simulink model "SpeedControlTest_vDemo_TC"  (Simulink 6.6)
settings: Solver=ode4  SolverMode=SingleTasking  StartTime=0.0  StopTime=252  FixedStep=0.01  RelTol=1e-3
InitFcn:
  | tempomat_para
StopFcn:
  | clear;
values from neighbouring files (symbols this model uses):
  A = 1.9    [tempomat_para.m]
  a_Fzg_max = 2    [tempomat_para.m]
  a_Fzg_min = -2    [tempomat_para.m]
  cw = 0.32    [tempomat_para.m]
  gang = [1 2 3 4]    [tempomat_para.m]
  gang_vec = [1 2 3 4]    [tempomat_para.m]
  i_anteil = 5    [tempomat_para.m]
  i_d = 3.42    [tempomat_para.m]
  i_g = [3.91 2.17 1.37 1.00]    [tempomat_para.m]
  lambda_gang = [1.3 1.25  1.17  1.05]    [tempomat_para.m]
  m_Fzg = 1400    [tempomat_para.m]
  M_mot_max = [130 149 163 170 168 166 162 158 150 139 123 80]    [tempomat_para.m]
  M_mot_min = [0 -40]    [tempomat_para.m]
  n_mot0 = 1000    [tempomat_para.m]
  n_mot_max = 1000:500:6500    [tempomat_para.m]
  n_mot_min = [1000 6500]    [tempomat_para.m]
  p_anteil = 100    [tempomat_para.m]
  r_dyn = 0.28    [tempomat_para.m]
  rho = 1.202    [tempomat_para.m]
  t_sch = 0.2    [tempomat_para.m]
  TI = [block '/TI']    [PSTI_callback.m]
  v_Fzg_ms0 = 0    [tempomat_para.m]
undefined symbols (not defined in the file or in its folder): Drossel_mat, getdatatypespecs
libraries: simulink x113, fzgbib x3
(part 3 of 9)

== system SpeedControlTest_vDemo_TC/Validation Functions/R1 Speed Control step response/Maximum overshoot < 5 &  Steady state error < 5/Step response characteristics ==
  Step : Inport
  Step response : Inport  Port=2
  Step response characteristics extraction : Subsystem  mask(Step response feature extraction){gain=1, lowerLim=10, upperLim=90, MOma=0.01*ones(1,100), RelTol=0.0001, MinTime=5, Range=5, sseW=0.01*ones(1,100)}
      mask prompts: gain "System's static gain"; lowerLim "Rise time interval lower limit (in set point %)"; upperLim "Rise time interval upper limit (in set point %)"; MOma "Maximum overshoot moving average weights"; RelTol "Maximum overshoot - Detect constant if no overshoot - Relative Tolerance"; MinTime "Maximum overshoot - Detect constant if no overshoot - Minimum constant time"; Range "Settling time range (in set point %)"; sseW "Steady state error - moving average weights"
      mask help: Extracts four step response feature characteristics. Extraction parameters are shown below.
      mask CallbackString:
      | set_param([gcb '/Static Gain'],'Value',get_param(gcb,'gain'));|set_param([gcb '/Extract rise time/lowerLim'],'Value',get_param(gcb,'lowerLim'));|set_param([gcb '/Extract rise time/upperLim'],'Value',get_param(gcb,'upperLim'));|set_param([gcb '/Extract maximum overshoot/Step response moving average and initial conditions before step/Weighted Moving Average'],'mgainval',get_param(gcb,'MOma'));
      | set_param([gcb '/Extract maximum overshoot/Step response moving average and initial conditions before step/Weighted Moving Average1'],'mgainval',get_param(gcb,'MOma'));|set_param([gcb '/Extract maximum overshoot/Active if signals constant for some specified time/Time since signal constant'],'RT',get_param(gcb,'RelTol'));
      | set_param([gcb '/Extract maximum overshoot/Active if signals constant for some specified time/Time since signal constant1'],'RT',get_param(gcb,'RelTol'));|set_param([gcb '/Extract maximum overshoot/Active if signals constant for some specified time/Min Time'],'Value',get_param(gcb,'MinTime'));|set_param([gcb '/Extract settling time/Set point percent'],'Value',get_param(gcb,'Range'));|set_param([gcb '/Extract steady state error/Weighted Moving Average'],'mgainval',get_param(gcb,'sseW'));
  Step response reset : Subsystem  mask{MT=10, RT=0.0001, MSS=10}
      mask prompts: MT "Minimal time for signals to be constant before a step"; RT "Relative tolerance for constant detection in %"; MSS "Minimal step size for step detection"
      mask CallbackString:
      | if (str2double(get_param(gcb,'MT')) < 0)
      |     error(['Minimal time specified (' get_param(gcb,'MT') ') negative. Please give a non-negative value.']);
      | else
      |     set_param([gcb '/Active if signals constant for some specified time/Min Time'],'Value',get_param(gcb,'MT'));
      | end|if or( (str2double(get_param(gcb,'RT')) < 0), (str2double(get_param(gcb,'RT')) > 100))
      |     error(['Relative tolerance value (' get_param(gcb,'RT') ') out of range. Please give a value between 0 and 100.']);
      | else
      |     set_param([gcb '/Active if signals constant for some specified time/Time since signal constant/Detect constant/Relative tolerance/Relative Tolerance'],'Value',get_param(gcb,'RT'));
      |     set_param([gcb '/Active if signals constant for some specified time/Time since signal constant/Detect constant'],'RT',get_param(gcb,'RT'));
      |     set_param([gcb '/Active if signals constant for some specified time/Time since signal constant'],'RT',get_param(gcb,'RT'));
      |     set_param([gcb '/Active if signals constant for some specified time/Time since signal constant1/Detect constant/Relative tolerance/Relative Tolerance'],'Value',get_param(gcb,'RT'));
      |     set_param([gcb '/Active if signals constant for some specified time/Time since signal constant1/Detect constant'],'RT',get_param(gcb,'RT'));
      |     set_param([gcb '/Active if signals constant for some specified time/Time since signal constant1'],'RT',get_param(gcb,'RT'));
      | end|if (str2double(get_param(gcb,'MSS')) < 0)
      |     error(['Minimal step size specified (' get_param(gcb,'MSS') ') negative. Please give a non-negative value.']);
      | else
      |     set_param([gcb '/Step detection/Min step size'],'Value',get_param(gcb,'MSS'));
      |     set_param([gcb '/Step detection'],'StepSize',get_param(gcb,'MSS'));
      | 
      | end
  Step response trigger : Subsystem  mask(Step response trigger extraction){MinTime=10, RelTol=0.001, MAXsse=5}
      mask prompts: MinTime "Detect constant signals - Minimum constant time"; RelTol "Detect constant signals - Relative Tolerance"; MAXsse "Maximum steady state error for triggering"
      mask help: This block extracts the trigger signals for the four step response characteristics.
      mask CallbackString:
      | set_param([gcb '/Active if signals constant for some specified time/Min Time'],'Value',get_param(gcb,'MinTime'));|set_param([gcb '/Active if signals constant for some specified time/Time since signal constant'],'RT',get_param(gcb,'RelTol'));
      | set_param([gcb '/Active if signals constant for some specified time/Time since signal constant1'],'RT',get_param(gcb,'RelTol'));|set_param([gcb '/Compare To Constant'],'const',get_param(gcb,'MAXsse'));
  R : Outport
  Rise time T : Outport  Port=2  DataType=double
  Overshoot T : Outport  Port=3  DataType=double
  Settling time T : Outport  Port=4  DataType=double
  Steady state error T : Outport  Port=5  DataType=double
  Rise time : Outport  Port=6
  Maximum Overshoot : Outport  Port=7
  Settling time : Outport  Port=8  DataType=double
  Steady state error : Outport  Port=9  DataType=double
  wires:
  Step response reset/1(R) -> R/1, Step response characteristics extraction/1(R)
  Step response characteristics extraction/4(Steady state error) -> Step response trigger/1(Steady state error), Steady state error/1
  Step/1 -> Step response reset/1(Step), Step response characteristics extraction/2(Step)
  Step response/1 -> Step response reset/2(Step response), Step response characteristics extraction/3(Step response), Step response trigger/2(Step response)
  Step response characteristics extraction/1(Rise time) -> Rise time/1
  Step response characteristics extraction/3(Settling time) -> Settling time/1
  Step response characteristics extraction/2(Maximum overshoot) -> Maximum Overshoot/1
  Step response trigger/1(Rise time T) -> Rise time T/1
  Step response trigger/2(Overshoot T) -> Overshoot T/1
  Step response trigger/3(Settling time T) -> Settling time T/1
  Step response trigger/4(Steady state error T) -> Steady state error T/1

== system SpeedControlTest_vDemo_TC/Validation Functions/R2 Speed Control velocity restoration time after simple  acceleration or deceleration/CC active + no target & Speed Control active & step of V_Des = |1|  with time periods >= 7s/CC active & no target ==
  Signal : Inport
  Reference : Inport  Port=2
  Abs : Abs
  Abs1 : Abs
  Absolute Tolerance : Constant  Value=AbsoluteTolerance
  Add : Sum  Inputs=+-  OutScaling=2^-10
  Relational Operator : RelationalOperator  Operator===  LogicOutDataTypeMode=Boolean
  Activate : Outport
  wires:
  Relational Operator/1 -> Activate/1
  Abs/1 -> Relational Operator/1
  Add/1 -> Abs/1
  Signal/1 -> Add/1
  Reference/1 -> Add/2
  Absolute Tolerance/1 -> Abs1/1
  Abs1/1 -> Relational Operator/2

== system SpeedControlTest_vDemo_TC/Validation Functions/R2 Speed Control velocity restoration time after simple  acceleration or deceleration/CC active + no target & Speed Control active & step of V_Des = |1|  with time periods >= 7s/CC active & no target1 ==
  Signal : Inport
  Reference : Inport  Port=2
  Abs : Abs
  Abs1 : Abs
  Absolute Tolerance : Constant  Value=AbsoluteTolerance
  Add : Sum  Inputs=+-  OutScaling=2^-10
  Relational Operator : RelationalOperator  Operator===  LogicOutDataTypeMode=Boolean
  Activate : Outport
  wires:
  Relational Operator/1 -> Activate/1
  Abs/1 -> Relational Operator/1
  Add/1 -> Abs/1
  Signal/1 -> Add/1
  Reference/1 -> Add/2
  Absolute Tolerance/1 -> Abs1/1
  Abs1/1 -> Relational Operator/2

== system SpeedControlTest_vDemo_TC/Validation Functions/R2 Speed Control velocity restoration time after simple  acceleration or deceleration/CC active + no target & Speed Control active & step of V_Des = |1|  with time periods >= 7s/PS ==
  A TI1 : Inport
  A TI2 : Inport  Port=2
  A TI3 : Inport  Port=3
  AND : Logic  Inputs=4  AllPortsSameDT=off  OutDataTypeMode=Boolean
  Bus Creator : BusCreator  Inputs=3
  Data Type Conversion : DataTypeConversion
  Data Type Conversion1 : DataTypeConversion
  Data Type Conversion2 : DataTypeConversion
  Max Delay A : Subsystem  TreatAsAtomicUnit=on  mask{Delay=0}
      mask prompts: Delay "Delay (in simulation steps) for the input signal:"
      mask init:
      | %set_param([gcb '/Discrete Transfer Fcn'],'Denominator',['[' num2str([1 zeros(1,str2double(get_param(gcb,'Delay')))]) ']']);
      mask CallbackString:
      | Delay = str2double(get_param(gcb,'Delay'));
      | if Delay < 0
      |     set_param(gcb,'Delay','0');
      |     error('Only non-negative delays are possible (causality).');
      |     set_param([gcb '/Delay'],'Value','0');
      | elseif Delay == 0
      |     set_param([gcb '/Delay'],'Value','0');
      | else
      |     set_param([gcb '/Integer Delay'],'NumDelays',num2str(Delay));
      |     set_param([gcb '/Delay'],'Value',num2str(Delay));
      | end
      mask Display: text(0.5,0.5,['z^{ ' num2str((-1)*str2double(get_param(gcb,'Delay'))) '}'],'texmode','on');
  Max Delay R : Subsystem  TreatAsAtomicUnit=on  mask{Delay=0}
      mask prompts: Delay "Delay (in simulation steps) for the input signal:"
      mask init:
      | %set_param([gcb '/Discrete Transfer Fcn'],'Denominator',['[' num2str([1 zeros(1,str2double(get_param(gcb,'Delay')))]) ']']);
      mask CallbackString:
      | Delay = str2double(get_param(gcb,'Delay'));
      | if Delay < 0
      |     set_param(gcb,'Delay','0');
      |     error('Only non-negative delays are possible (causality).');
      |     set_param([gcb '/Delay'],'Value','0');
      | elseif Delay == 0
      |     set_param([gcb '/Delay'],'Value','0');
      | else
      |     set_param([gcb '/Integer Delay'],'NumDelays',num2str(Delay));
      |     set_param([gcb '/Delay'],'Value',num2str(Delay));
      | end
      mask Display: text(0.5,0.5,['z^{ ' num2str((-1)*str2double(get_param(gcb,'Delay'))) '}'],'texmode','on');
  Max Delay T : Subsystem  TreatAsAtomicUnit=on  mask{Delay=0}
      mask prompts: Delay "Delay (in simulation steps) for the input signal:"
      mask init:
      | %set_param([gcb '/Discrete Transfer Fcn'],'Denominator',['[' num2str([1 zeros(1,str2double(get_param(gcb,'Delay')))]) ']']);
      mask CallbackString:
      | Delay = str2double(get_param(gcb,'Delay'));
      | if Delay < 0
      |     set_param(gcb,'Delay','0');
      |     error('Only non-negative delays are possible (causality).');
      |     set_param([gcb '/Delay'],'Value','0');
      | elseif Delay == 0
      |     set_param([gcb '/Delay'],'Value','0');
      | else
      |     set_param([gcb '/Integer Delay'],'NumDelays',num2str(Delay));
      |     set_param([gcb '/Delay'],'Value',num2str(Delay));
      | end
      mask Display: text(0.5,0.5,['z^{ ' num2str((-1)*str2double(get_param(gcb,'Delay'))) '}'],'texmode','on');
  OR - AND : Subsystem
  TDD : Subsystem
  TI : Subsystem
  TID : Subsystem
  Precond : Outport
  wires:
  Data Type Conversion2/1 -> Bus Creator/3  "R"
  TI/1(A) -> AND/2
  OR - AND/1(OR) -> TID/1(R OR)
  OR - AND/2(AND) -> Max Delay R/1(In1), TID/2(R AND)
  AND/1 -> Data Type Conversion2/1
  Max Delay A/1(Out1) -> Data Type Conversion/1
  Max Delay R/1(Out1) -> AND/1
  Max Delay T/1(Out1) -> Data Type Conversion1/1
  TDD/1(A) -> AND/3
  Data Type Conversion1/1 -> Bus Creator/2  "T"
  Data Type Conversion/1 -> Bus Creator/1  "A"
  Bus Creator/1 -> Precond/1
  TID/1(A) -> Max Delay A/1(In1)
  TID/2(T) -> Max Delay T/1(In1)
  TDD/2(T) -> AND/4
  A TI1/1 -> TI/1(A1)
  A TI2/1 -> TI/2(A2)
  A TI3/1 -> TI/3(A3)

== system SpeedControlTest_vDemo_TC/Validation Functions/R2 Speed Control velocity restoration time after simple  acceleration or deceleration/CC active + no target & Speed Control active & step of V_Des = |1|  with time periods >= 7s/Speed control active ==
  Signal : Inport
  Reference : Inport  Port=2
  Abs : Abs
  Abs1 : Abs
  Absolute Tolerance : Constant  Value=AbsoluteTolerance
  Add : Sum  Inputs=+-  OutScaling=2^-10
  Relational Operator : RelationalOperator  Operator===  LogicOutDataTypeMode=Boolean
  Activate : Outport
  wires:
  Abs1/1 -> Relational Operator/2
  Absolute Tolerance/1 -> Abs1/1
  Reference/1 -> Add/2
  Signal/1 -> Add/1
  Add/1 -> Abs/1
  Abs/1 -> Relational Operator/1
  Relational Operator/1 -> Activate/1

== system SpeedControlTest_vDemo_TC/Validation Functions/R2 Speed Control velocity restoration time after simple  acceleration or deceleration/CC active + no target & Speed Control active & step of V_Des = |1|  with time periods >= 7s/Step with step size=|1|  and time periods >= 6s detection ==
  Step : Inport
  Step detection : Subsystem  mask{MT=6, RT=0.0001, MSS=1}
      mask prompts: MT "Minimal time for signals to be constant before a step"; RT "Relative tolerance for constant detection in %"; MSS "Step size for step detection"
      mask CallbackString:
      | if (str2double(get_param(gcb,'MT')) < 0)
      |     error(['Minimal time specified (' get_param(gcb,'MT') ') negative. Please give a non-negative value.']);
      | else
      |     set_param([gcb '/Active if signals constant for some specified time/Min Time'],'Value',get_param(gcb,'MT'));
      | end|if or( (str2double(get_param(gcb,'RT')) < 0), (str2double(get_param(gcb,'RT')) > 100))
      |     error(['Relative tolerance value (' get_param(gcb,'RT') ') out of range. Please give a value between 0 and 100.']);
      | else
      |     set_param([gcb '/Active if signals constant for some specified time/Time since signal constant1/Detect constant/Relative tolerance/Relative Tolerance'],'Value',get_param(gcb,'RT'));
      |     set_param([gcb '/Active if signals constant for some specified time/Time since signal constant1/Detect constant'],'RT',get_param(gcb,'RT'));
      |     set_param([gcb '/Active if signals constant for some specified time/Time since signal constant1'],'RT',get_param(gcb,'RT'));
      | end|if (str2double(get_param(gcb,'MSS')) < 0)
      |     error(['Step size specified (' get_param(gcb,'MSS') ') negative. Please give a non-negative value.']);
      | else
      |     set_param([gcb '/Step detection/Step size'],'Value',get_param(gcb,'MSS'));
      |     set_param([gcb '/Step detection'],'StepSize',get_param(gcb,'MSS'));
      | 
      | end
  Complete step : Outport
  wires:
  Step/1 -> Step detection/1(Step)
  Step detection/1(R) -> Complete step/1

== system SpeedControlTest_vDemo_TC/Validation Functions/R2 Speed Control velocity restoration time after simple  acceleration or deceleration/after (6 seconds)  |V_Des-V_Vhcl <= 1.4|/  ==
  Signal : Inport
  Reference : Inport  Port=2
  Bus Creator : BusCreator  Inputs=5
  Data Type Conversion{,1..3} (4 alike) : DataTypeConversion
  Delay : Constant  Value=0
  LOWER : Constant  Value=Lower  OutDataTypeMode=int8
  No Limit : Constant  Value=Inf
  No limit : Constant  Value=-Inf
  Relational Operator : RelationalOperator  Operator=<=  LogicOutDataTypeMode=Boolean  LogicDataType=double
  Switch 2 : Switch  Criteria=u2 ~= 0
  Switch 3 : Switch  Criteria=u2 ~= 0
  UPPER : Constant  Value=Upper  OutDataTypeMode=int8
  V : Outport  InitialOutput=[2]
  wires:
  Relational Operator/1 -> Data Type Conversion/1
  Data Type Conversion3/1 -> Bus Creator/4  "Actual data"
  Data Type Conversion2/1 -> Bus Creator/3  "Expected upper limit"
  Data Type Conversion1/1 -> Bus Creator/2  "Expected lower limit"
  Data Type Conversion/1 -> Bus Creator/1  "Local verdict"
  Bus Creator/1 -> V/1
  Reference/1 -> Relational Operator/2, Switch 2/3, Switch 3/3
  Signal/1 -> Data Type Conversion3/1, Relational Operator/1
  UPPER/1 -> Switch 3/2
  No Limit/1 -> Switch 3/1
  LOWER/1 -> Switch 2/2
  No limit/1 -> Switch 2/1
  Switch 2/1 -> Data Type Conversion1/1
  Switch 3/1 -> Data Type Conversion2/1
  Delay/1 -> Bus Creator/5  "Delay"

== system SpeedControlTest_vDemo_TC/Validation Functions/R2 Speed Control velocity restoration time after simple  acceleration or deceleration/after (6 seconds)  |V_Des-V_Vhcl <= 1.4|/PAS1 ==
  Precond : Inport
  V : Inport  Port=2
  A delay : Subsystem  TreatAsAtomicUnit=on  mask{Delay=600}
      mask prompts: Delay "Delay (in simulation steps) for the input signal:"
      mask init:
      | %set_param([gcb '/Discrete Transfer Fcn'],'Denominator',['[' num2str([1 zeros(1,str2double(get_param(gcb,'Delay')))]) ']']);
      mask CallbackString:
      | Delay = str2double(get_param(gcb,'Delay'));
      | if Delay < 0
      |     set_param(gcb,'Delay','0');
      |     error('Only non-negative delays are possible (causality).');
      |     set_param([gcb '/Delay'],'Value','0');
      | elseif Delay == 0
      |     set_param([gcb '/Delay'],'Value','0');
      | else
      |     set_param([gcb '/Integer Delay'],'NumDelays',num2str(Delay));
      |     set_param([gcb '/Delay'],'Value',num2str(Delay));
      | end
      mask Display: text(0.5,0.5,['z^{ ' num2str((-1)*str2double(get_param(gcb,'Delay'))) '}'],'texmode','on');
  AND1 : Logic  AllPortsSameDT=off  OutDataTypeMode=Boolean
  Bus Selector : BusSelector  OutputSignals=Local verdict
  Bus Selector1 : BusSelector  OutputSignals=Expected lower limit,Expected upper limit,Actual data
  Bus Selector2 : BusSelector  OutputSignals=R,T,A
  Bus Assignment : BusAssignment  AssignedSignals=Local verdict,Delay
  Bus Assignment1 : BusAssignment  AssignedSignals=Expected lower limit,Expected upper limit,Actual data
  Constant : Constant  Value=-1
  Delay bus signals : Subsystem
  Ra delay : Subsystem  TreatAsAtomicUnit=on  mask{Delay=0}
      mask prompts: Delay "Delay (in simulation steps) for the input signal:"
      mask init:
      | %set_param([gcb '/Discrete Transfer Fcn'],'Denominator',['[' num2str([1 zeros(1,str2double(get_param(gcb,'Delay')))]) ']']);
      mask CallbackString:
      | Delay = str2double(get_param(gcb,'Delay'));
      | if Delay < 0
      |     set_param(gcb,'Delay','0');
      |     error('Only non-negative delays are possible (causality).');
      |     set_param([gcb '/Delay'],'Value','0');
      | elseif Delay == 0
      |     set_param([gcb '/Delay'],'Value','0');
      | else
      |     set_param([gcb '/Integer Delay'],'NumDelays',num2str(Delay));
      |     set_param([gcb '/Delay'],'Value',num2str(Delay));
      | end
      mask Display: text(0.5,0.5,['z^{ ' num2str((-1)*str2double(get_param(gcb,'Delay'))) '}'],'texmode','on');
  Rp delay : Subsystem  TreatAsAtomicUnit=on  mask{Delay=600}
      mask prompts: Delay "Delay (in simulation steps) for the input signal:"
      mask init:
      | %set_param([gcb '/Discrete Transfer Fcn'],'Denominator',['[' num2str([1 zeros(1,str2double(get_param(gcb,'Delay')))]) ']']);
      mask CallbackString:
      | Delay = str2double(get_param(gcb,'Delay'));
      | if Delay < 0
      |     set_param(gcb,'Delay','0');
      |     error('Only non-negative delays are possible (causality).');
      |     set_param([gcb '/Delay'],'Value','0');
      | elseif Delay == 0
      |     set_param([gcb '/Delay'],'Value','0');
      | else
      |     set_param([gcb '/Integer Delay'],'NumDelays',num2str(Delay));
      |     set_param([gcb '/Delay'],'Value',num2str(Delay));
      | end
      mask Display: text(0.5,0.5,['z^{ ' num2str((-1)*str2double(get_param(gcb,'Delay'))) '}'],'texmode','on');
  Ta delay : Subsystem  TreatAsAtomicUnit=on  mask{Delay=0}
      mask prompts: Delay "Delay (in simulation steps) for the input signal:"
      mask init:
      | %set_param([gcb '/Discrete Transfer Fcn'],'Denominator',['[' num2str([1 zeros(1,str2double(get_param(gcb,'Delay')))]) ']']);
      mask CallbackString:
      | Delay = str2double(get_param(gcb,'Delay'));
      | if Delay < 0
      |     set_param(gcb,'Delay','0');
      |     error('Only non-negative delays are possible (causality).');
      |     set_param([gcb '/Delay'],'Value','0');
      | elseif Delay == 0
      |     set_param([gcb '/Delay'],'Value','0');
      | else
      |     set_param([gcb '/Integer Delay'],'NumDelays',num2str(Delay));
      |     set_param([gcb '/Delay'],'Value',num2str(Delay));
      | end
      mask Display: text(0.5,0.5,['z^{ ' num2str((-1)*str2double(get_param(gcb,'Delay'))) '}'],'texmode','on');
  Tp delay : Subsystem  TreatAsAtomicUnit=on  mask{Delay=600}
      mask prompts: Delay "Delay (in simulation steps) for the input signal:"
      mask init:
      | %set_param([gcb '/Discrete Transfer Fcn'],'Denominator',['[' num2str([1 zeros(1,str2double(get_param(gcb,'Delay')))]) ']']);
      mask CallbackString:
      | Delay = str2double(get_param(gcb,'Delay'));
      | if Delay < 0
      |     set_param(gcb,'Delay','0');
      |     error('Only non-negative delays are possible (causality).');
      |     set_param([gcb '/Delay'],'Value','0');
      | elseif Delay == 0
      |     set_param([gcb '/Delay'],'Value','0');
      | else
      |     set_param([gcb '/Integer Delay'],'NumDelays',num2str(Delay));
      |     set_param([gcb '/Delay'],'Value',num2str(Delay));
      | end
      mask Display: text(0.5,0.5,['z^{ ' num2str((-1)*str2double(get_param(gcb,'Delay'))) '}'],'texmode','on');
  V delay : Subsystem  TreatAsAtomicUnit=on  mask{Delay=0}
      mask prompts: Delay "Delay (in simulation steps) for the input signal:"
      mask init:
      | %set_param([gcb '/Discrete Transfer Fcn'],'Denominator',['[' num2str([1 zeros(1,str2double(get_param(gcb,'Delay')))]) ']']);
      mask CallbackString:
      | Delay = str2double(get_param(gcb,'Delay'));
      | if Delay < 0
      |     set_param(gcb,'Delay','0');
      |     error('Only non-negative delays are possible (causality).');
      |     set_param([gcb '/Delay'],'Value','0');
      | elseif Delay == 0
      |     set_param([gcb '/Delay'],'Value','0');
      | else
      |     set_param([gcb '/Integer Delay'],'NumDelays',num2str(Delay));
      |     set_param([gcb '/Delay'],'Value',num2str(Delay));
      | end
      mask Display: text(0.5,0.5,['z^{ ' num2str((-1)*str2double(get_param(gcb,'Delay'))) '}'],'texmode','on');
  error : Subsystem
  none - pass - fail : Subsystem
  sw D : Switch  Criteria=u2 ~= 0
  sw V : Switch  Criteria=u2 ~= 0
  VF Info : Outport
  wires:
  Ta delay/1(Out1) -> error/5(Ta), none - pass - fail/5(Ta)
  Delay bus signals/3(ADout) -> Bus Assignment1/4
  Delay bus signals/2(EULout) -> Bus Assignment1/3
  Delay bus signals/1(ELLout) -> Bus Assignment1/2
  Bus Assignment1/1 -> Bus Assignment/1
  Bus Selector1/3 -> Delay bus signals/3(ADin)  "<Actual data>"
  Bus Selector1/2 -> Delay bus signals/2(EULin)  "<Expected upper limit>"
  Bus Selector1/1 -> Delay bus signals/1(ELLin)  "<Expected lower limit>"
  Precond/1 -> Bus Selector2/1
  AND1/1 -> none - pass - fail/7(R AND)
  Ra delay/1(Out1) -> error/4(Ra), AND1/2, none - pass - fail/4(Ra)
  V delay/1(Out1) -> none - pass - fail/6(V), error/6(V)
  A delay/1(Out1) -> none - pass - fail/3(A), error/3(A)
  Tp delay/1(Out1) -> none - pass - fail/2(Tp), error/2(Tp)
  Rp delay/1(Out1) -> AND1/1, none - pass - fail/1(Rp), error/1(Rp)
  Bus Selector2/3 -> A delay/1(In1)  "<A>"
  Bus Selector2/2 -> Tp delay/1(In1)  "<T>"
  Bus Selector2/1 -> Rp delay/1(In1)  "<R>"
  Bus Assignment/1 -> VF Info/1
  Bus Selector/1 -> V delay/1(In1), Ta delay/1(In1), Ra delay/1(In1)  "<Local verdict>"
  sw D/1 -> Bus Assignment/3
  sw V/1 -> Bus Assignment/2
  none - pass - fail/3(Delay) -> sw D/3
  none - pass - fail/2(MaxDelay) -> sw D/1
  none - pass - fail/1(Verdict) -> sw V/3
  Constant/1 -> sw V/1
  error/1(Verror) -> sw D/2, sw V/2
  V/1 -> Bus Assignment1/1, Bus Selector1/1, Bus Selector/1

== system SpeedControlTest_vDemo_TC/Validation Functions/R2 Speed Control velocity restoration time after simple  acceleration or deceleration/after (6 seconds)  |V_Des-V_Vhcl <= 1.4|/PAS2 ==
  Precond : Inport
  V : Inport  Port=2
  A delay : Subsystem  TreatAsAtomicUnit=on  mask{Delay=600}
      mask prompts: Delay "Delay (in simulation steps) for the input signal:"
      mask init:
      | %set_param([gcb '/Discrete Transfer Fcn'],'Denominator',['[' num2str([1 zeros(1,str2double(get_param(gcb,'Delay')))]) ']']);
      mask CallbackString:
      | Delay = str2double(get_param(gcb,'Delay'));
      | if Delay < 0
      |     set_param(gcb,'Delay','0');
      |     error('Only non-negative delays are possible (causality).');
      |     set_param([gcb '/Delay'],'Value','0');
      | elseif Delay == 0
      |     set_param([gcb '/Delay'],'Value','0');
      | else
      |     set_param([gcb '/Integer Delay'],'NumDelays',num2str(Delay));
      |     set_param([gcb '/Delay'],'Value',num2str(Delay));
      | end
      mask Display: text(0.5,0.5,['z^{ ' num2str((-1)*str2double(get_param(gcb,'Delay'))) '}'],'texmode','on');
  AND1 : Logic  AllPortsSameDT=off  OutDataTypeMode=Boolean
  Bus Selector : BusSelector  OutputSignals=Local verdict
  Bus Selector1 : BusSelector  OutputSignals=Expected lower limit,Expected upper limit,Actual data
  Bus Selector2 : BusSelector  OutputSignals=R,T,A
  Bus Assignment : BusAssignment  AssignedSignals=Local verdict,Delay
  Bus Assignment1 : BusAssignment  AssignedSignals=Expected lower limit,Expected upper limit,Actual data
  Constant : Constant  Value=-1
  Delay bus signals : Subsystem
  Ra delay : Subsystem  TreatAsAtomicUnit=on  mask{Delay=0}
      mask prompts: Delay "Delay (in simulation steps) for the input signal:"
      mask init:
      | %set_param([gcb '/Discrete Transfer Fcn'],'Denominator',['[' num2str([1 zeros(1,str2double(get_param(gcb,'Delay')))]) ']']);
      mask CallbackString:
      | Delay = str2double(get_param(gcb,'Delay'));
      | if Delay < 0
      |     set_param(gcb,'Delay','0');
      |     error('Only non-negative delays are possible (causality).');
      |     set_param([gcb '/Delay'],'Value','0');
      | elseif Delay == 0
      |     set_param([gcb '/Delay'],'Value','0');
      | else
      |     set_param([gcb '/Integer Delay'],'NumDelays',num2str(Delay));
      |     set_param([gcb '/Delay'],'Value',num2str(Delay));
      | end
      mask Display: text(0.5,0.5,['z^{ ' num2str((-1)*str2double(get_param(gcb,'Delay'))) '}'],'texmode','on');
  Rp delay : Subsystem  TreatAsAtomicUnit=on  mask{Delay=600}
      mask prompts: Delay "Delay (in simulation steps) for the input signal:"
      mask init:
      | %set_param([gcb '/Discrete Transfer Fcn'],'Denominator',['[' num2str([1 zeros(1,str2double(get_param(gcb,'Delay')))]) ']']);
      mask CallbackString:
      | Delay = str2double(get_param(gcb,'Delay'));
      | if Delay < 0
      |     set_param(gcb,'Delay','0');
      |     error('Only non-negative delays are possible (causality).');
      |     set_param([gcb '/Delay'],'Value','0');
      | elseif Delay == 0
      |     set_param([gcb '/Delay'],'Value','0');
      | else
      |     set_param([gcb '/Integer Delay'],'NumDelays',num2str(Delay));
      |     set_param([gcb '/Delay'],'Value',num2str(Delay));
      | end
      mask Display: text(0.5,0.5,['z^{ ' num2str((-1)*str2double(get_param(gcb,'Delay'))) '}'],'texmode','on');
  Ta delay : Subsystem  TreatAsAtomicUnit=on  mask{Delay=0}
      mask prompts: Delay "Delay (in simulation steps) for the input signal:"
      mask init:
      | %set_param([gcb '/Discrete Transfer Fcn'],'Denominator',['[' num2str([1 zeros(1,str2double(get_param(gcb,'Delay')))]) ']']);
      mask CallbackString:
      | Delay = str2double(get_param(gcb,'Delay'));
      | if Delay < 0
      |     set_param(gcb,'Delay','0');
      |     error('Only non-negative delays are possible (causality).');
      |     set_param([gcb '/Delay'],'Value','0');
      | elseif Delay == 0
      |     set_param([gcb '/Delay'],'Value','0');
      | else
      |     set_param([gcb '/Integer Delay'],'NumDelays',num2str(Delay));
      |     set_param([gcb '/Delay'],'Value',num2str(Delay));
      | end
      mask Display: text(0.5,0.5,['z^{ ' num2str((-1)*str2double(get_param(gcb,'Delay'))) '}'],'texmode','on');
  Tp delay : Subsystem  TreatAsAtomicUnit=on  mask{Delay=600}
      mask prompts: Delay "Delay (in simulation steps) for the input signal:"
      mask init:
      | %set_param([gcb '/Discrete Transfer Fcn'],'Denominator',['[' num2str([1 zeros(1,str2double(get_param(gcb,'Delay')))]) ']']);
      mask CallbackString:
      | Delay = str2double(get_param(gcb,'Delay'));
      | if Delay < 0
      |     set_param(gcb,'Delay','0');
      |     error('Only non-negative delays are possible (causality).');
      |     set_param([gcb '/Delay'],'Value','0');
      | elseif Delay == 0
      |     set_param([gcb '/Delay'],'Value','0');
      | else
      |     set_param([gcb '/Integer Delay'],'NumDelays',num2str(Delay));
      |     set_param([gcb '/Delay'],'Value',num2str(Delay));
      | end
      mask Display: text(0.5,0.5,['z^{ ' num2str((-1)*str2double(get_param(gcb,'Delay'))) '}'],'texmode','on');
  V delay : Subsystem  TreatAsAtomicUnit=on  mask{Delay=0}
      mask prompts: Delay "Delay (in simulation steps) for the input signal:"
      mask init:
      | %set_param([gcb '/Discrete Transfer Fcn'],'Denominator',['[' num2str([1 zeros(1,str2double(get_param(gcb,'Delay')))]) ']']);
      mask CallbackString:
      | Delay = str2double(get_param(gcb,'Delay'));
      | if Delay < 0
      |     set_param(gcb,'Delay','0');
      |     error('Only non-negative delays are possible (causality).');
      |     set_param([gcb '/Delay'],'Value','0');
      | elseif Delay == 0
      |     set_param([gcb '/Delay'],'Value','0');
      | else
      |     set_param([gcb '/Integer Delay'],'NumDelays',num2str(Delay));
      |     set_param([gcb '/Delay'],'Value',num2str(Delay));
      | end
      mask Display: text(0.5,0.5,['z^{ ' num2str((-1)*str2double(get_param(gcb,'Delay'))) '}'],'texmode','on');
  error : Subsystem
  none - pass - fail : Subsystem
  sw D : Switch  Criteria=u2 ~= 0
  sw V : Switch  Criteria=u2 ~= 0
  VF Info : Outport
  wires:
  Ta delay/1(Out1) -> error/5(Ta), none - pass - fail/5(Ta)
  Delay bus signals/3(ADout) -> Bus Assignment1/4
  Delay bus signals/2(EULout) -> Bus Assignment1/3
  Delay bus signals/1(ELLout) -> Bus Assignment1/2
  Bus Assignment1/1 -> Bus Assignment/1
  Bus Selector1/3 -> Delay bus signals/3(ADin)  "<Actual data>"
  Bus Selector1/2 -> Delay bus signals/2(EULin)  "<Expected upper limit>"
  Bus Selector1/1 -> Delay bus signals/1(ELLin)  "<Expected lower limit>"
  Precond/1 -> Bus Selector2/1
  AND1/1 -> none - pass - fail/7(R AND)
  Ra delay/1(Out1) -> error/4(Ra), AND1/2, none - pass - fail/4(Ra)
  V delay/1(Out1) -> none - pass - fail/6(V), error/6(V)
  A delay/1(Out1) -> none - pass - fail/3(A), error/3(A)
  Tp delay/1(Out1) -> none - pass - fail/2(Tp), error/2(Tp)
  Rp delay/1(Out1) -> AND1/1, none - pass - fail/1(Rp), error/1(Rp)
  Bus Selector2/3 -> A delay/1(In1)  "<A>"
  Bus Selector2/2 -> Tp delay/1(In1)  "<T>"
  Bus Selector2/1 -> Rp delay/1(In1)  "<R>"
  Bus Assignment/1 -> VF Info/1
  Bus Selector/1 -> V delay/1(In1), Ta delay/1(In1), Ra delay/1(In1)  "<Local verdict>"
  sw D/1 -> Bus Assignment/3
  sw V/1 -> Bus Assignment/2
  none - pass - fail/3(Delay) -> sw D/3
  none - pass - fail/2(MaxDelay) -> sw D/1
  none - pass - fail/1(Verdict) -> sw V/3
  Constant/1 -> sw V/1
  error/1(Verror) -> sw D/2, sw V/2
  V/1 -> Bus Assignment1/1, Bus Selector1/1, Bus Selector/1

== system SpeedControlTest_vDemo_TC/Validation Functions/R2 Speed Control velocity restoration time after simple  acceleration or deceleration/after (6 seconds)  |V_Des-V_Vhcl <= 1.4|/R = 2 ==
  In1 : Inport
  In2 : Inport  Port=2
  Abs1 : Abs
  "Active for  6s after R=1 " : Subsystem
  Bus Selector1 : BusSelector  OutputSignals=Outputs.v_Vhcl
  Hold1 : Subsystem  TreatAsAtomicUnit=on
      mask Display: patch(-0.31+[0.4 0.46 0.46 0.54 0.54 0.6 0.6 0.55 0.55 0.45 0.45 0.4],-0.19+[0.85 0.85 0.95 0.95 0.85 0.85 0.87 0.87 0.96 0.96 0.87 0.87],[0 0 0]);
  Hold2 : Subsystem  TreatAsAtomicUnit=on
      mask Display: patch(-0.31+[0.4 0.46 0.46 0.54 0.54 0.6 0.6 0.55 0.55 0.45 0.45 0.4],-0.19+[0.85 0.85 0.95 0.95 0.85 0.85 0.87 0.87 0.96 0.96 0.87 0.87],[0 0 0]);
  Minus1 : Sum  Inputs=+-  OutScaling=2^-10
  R = 1 : Subsystem
  Scope : Scope  NumInputPorts=5
      settings: YMin=-5~-5~-5~80~0  YMax=5~5~5~107.5~110  SaveName=ScopeData12  MaxDataPoints=5000000
  Out1 : Outport
  wires:
  In1/1 -> R = 1/1(In1), "Active for  6s after R=1 "/1(Signal 2)
  Hold1/1("  ") -> Minus1/1
  R = 1/1(Out1) -> Hold1/1(" "), Scope/2
  In2/1 -> Bus Selector1/1
  Bus Selector1/1 -> Hold1/2("    "), Hold2/2("    ")  "<v_Vhcl>"
  Hold2/1("  ") -> Minus1/2
  "Active for  6s after R=1 "/1(6s after) -> Hold2/1(" "), Scope/1
  Minus1/1 -> Abs1/1
  Abs1/1 -> Out1/1, Scope/3

== system SpeedControlTest_vDemo_TC/Validation Functions/R2 Speed Control velocity restoration time after simple  acceleration or deceleration/after (6 seconds)  |V_Des-V_Vhcl <= 1.4|/within(20 sec)1 ==
  Signal : Inport
  Reference : Inport  Port=2
  Bus Creator : BusCreator  Inputs=5
  Data Type Conversion{,1..3} (4 alike) : DataTypeConversion
  Delay : Constant  Value=0
  LOWER : Constant  Value=Lower  OutDataTypeMode=int8
  No Limit : Constant  Value=Inf
  No limit : Constant  Value=-Inf
  Relational Operator : RelationalOperator  Operator=<=  LogicOutDataTypeMode=Boolean  LogicDataType=double
  Switch 2 : Switch  Criteria=u2 ~= 0
  Switch 3 : Switch  Criteria=u2 ~= 0
  UPPER : Constant  Value=Upper  OutDataTypeMode=int8
  V : Outport  InitialOutput=[2]
  wires:
  Relational Operator/1 -> Data Type Conversion/1
  Data Type Conversion3/1 -> Bus Creator/4  "Actual data"
  Data Type Conversion2/1 -> Bus Creator/3  "Expected upper limit"
  Data Type Conversion1/1 -> Bus Creator/2  "Expected lower limit"
  Data Type Conversion/1 -> Bus Creator/1  "Local verdict"
  Bus Creator/1 -> V/1
  Reference/1 -> Relational Operator/2, Switch 2/3, Switch 3/3
  Signal/1 -> Data Type Conversion3/1, Relational Operator/1
  UPPER/1 -> Switch 3/2
  No Limit/1 -> Switch 3/1
  LOWER/1 -> Switch 2/2
  No limit/1 -> Switch 2/1
  Switch 2/1 -> Data Type Conversion1/1
  Switch 3/1 -> Data Type Conversion2/1
  Delay/1 -> Bus Creator/5  "Delay"

== system SpeedControlTest_vDemo_TC/Validation Functions/R2 Speed Control velocity restoration time after simple  acceleration or deceleration/after (6 seconds)  |V_Des-V_Vhcl <= 1.4|/|V_Des-V_Vhcl| ==
  InOut Bus : Inport
  Abs1 : Abs
  Bus Selector : BusSelector  OutputSignals=Inputs.v_Des,Outputs.v_Vhcl
  Minus1 : Sum  Inputs=+-  OutScaling=2^-10
  Out1 : Outport
  wires:
  Abs1/1 -> Out1/1
  Minus1/1 -> Abs1/1
  Bus Selector/2 -> Minus1/2  "<v_Vhcl>"
  InOut Bus/1 -> Bus Selector/1
  Bus Selector/1 -> Minus1/1  "<v_Des>"

== system SpeedControlTest_vDemo_TC/Speed control/Vehicle model/Fahrzeugmodell/Fahrwiderstaende/Schaltdauer ==
  note: 14.5.1996 Dieter Hoetzer / letzte aenderung
  note: Eine Wunschgangaenderung wird registriert und der neue Wunschgang solange im Speicher abgelegt,
      | bis die Schlatung beendet ist.
  Gang_w : Inport
  Memory1 : Memory  X0=1
  Relational Operator1 : RelationalOperator  Operator=~=  InputSameDT=on
  Schaltdauer : TransportDelay  DelayTime=t_sch  InitialOutput=1
  Speicher : Memory  X0=1
  Switch : Switch  Threshold=0.5  SaturateOnIntegerOverflow=on  InputSameDT=on
  ungleich : RelationalOperator  Operator=~=  InputSameDT=on
  k_l : Outport  InitialOutput=0
  wires:
  Relational Operator1/1 -> k_l/1
  Schaltdauer/1 -> Relational Operator1/2
  Speicher/1 -> Schaltdauer/1, Relational Operator1/1, Switch/3
  ungleich/1 -> Switch/2
  Memory1/1 -> ungleich/2
  Gang_w/1 -> Memory1/1, Switch/1, ungleich/1
  Switch/1 -> Speicher/1

== system SpeedControlTest_vDemo_TC/Speed control/Vehicle model/Fahrzeugmodell/Fahrzeugdynamik/Band-Limited White Noise ==
  Gain : Gain  Gain=[sqrt(Cov)]/[sqrt(Ts)]  SaturateOnIntegerOverflow=on
  White Noise : RandomNumber  Seed=seed
  Zero-Order Hold : ZeroOrderHold  SampleTime=Ts
  Out_1 : Outport  InitialOutput=0
  wires:
  White Noise/1 -> Zero-Order Hold/1
  Gain/1 -> Out_1/1
  Zero-Order Hold/1 -> Gain/1

== system SpeedControlTest_vDemo_TC/TestData 1/R1 Speed Control step response/Complete step & CC active + no target & Speed Control active/Generate complete step 5/Hold Time ==
  Clock : Inport
  Enable : EnablePort
  Write : DataStoreWrite  DataStoreName=triggerTime  SampleTime=-1
  wires:
  Clock/1 -> Write/1

== system SpeedControlTest_vDemo_TC/TestData 1/R1 Speed Control step response/Complete step & CC active + no target & Speed Control active/Generate complete step 5/Hold Value ==
  In1 : Inport
  Enable : EnablePort
  v_Des : Outport
  wires:
  In1/1 -> v_Des/1

== system SpeedControlTest_vDemo_TC/Validation Functions/R1 Speed Control step response/Complete step & CC active + no target & Speed Control active/Complete step detection/Step detection ==
  R : Inport
  Step : Inport  Port=2
  Step response : Inport  Port=3
  Active if signals constant for some specified time : Subsystem
  Detect constant : Subsystem  TreatAsAtomicUnit=on  mask(Feature extraction block){RT=0.0001}
      mask prompts: RT "Relative tolerance in %"
      mask help: Detect if the signal value is constant (using the last two signal values) allowing for a user-defined relative deviation
      mask CallbackString:
      | if or( (str2double(get_param(gcb,'RT')) < 0), (str2double(get_param(gcb,'RT')) > 100))
      |     error(['Relative tolerance value (' get_param(gcb,'RT') ') out of range. Please give a value between 0 and 100.']);
      | else
      |     set_param([gcb '/Relative tolerance/Relative Tolerance'],'Value',get_param(gcb,'RT'));
      | end
  Detect decrease : Subsystem  TreatAsAtomicUnit=on  mask(Detect increase){Param=0}
      mask prompts: Param "Mask Parameter 1:"
  Detect increase : Subsystem  TreatAsAtomicUnit=on  mask(Detect increase){Param=0}
      mask prompts: Param "Mask Parameter 1:"
  Detect increase2 : Subsystem  TreatAsAtomicUnit=on  mask(Detect increase){Param=0}
      mask prompts: Param "Mask Parameter 1:"
  Hold1 : Subsystem  TreatAsAtomicUnit=on
      mask Display: patch(-0.31+[0.4 0.46 0.46 0.54 0.54 0.6 0.6 0.55 0.55 0.45 0.45 0.4],-0.19+[0.85 0.85 0.95 0.95 0.85 0.85 0.87 0.87 0.96 0.96 0.87 0.87],[0 0 0]);
  Logical Operator : Logic  AllPortsSameDT=off  OutDataTypeMode=Boolean
  Logical Operator1 : Logic  Operator=NOT  AllPortsSameDT=off  OutDataTypeMode=Boolean
  Logical Operator2 : Logic  Operator=OR  Inputs=3  AllPortsSameDT=off  OutDataTypeMode=Boolean
  Memory2 : Memory
  End of complete step : Outport
  wires:
  Detect increase/1(Increase) -> Logical Operator2/1
  Detect constant/1(Constant) -> Logical Operator1/1
  Detect decrease/1(Decrease) -> Logical Operator2/2
  Logical Operator2/1 -> Hold1/1(" ")
  R/1 -> Hold1/2("    ")
  Step/1 -> Active if signals constant for some specified time/1(Signal1), Detect constant/1(Signal)
  Step response/1 -> Active if signals constant for some specified time/2(Signal 2)
  Active if signals constant for some specified time/1(Constant signals) -> Detect decrease/1(Signal), Detect increase/1(Signal), Detect increase2/1(Signal)
  Hold1/1("  ") -> Memory2/1
  Logical Operator/1 -> End of complete step/1
  Memory2/1 -> Logical Operator/2
  Detect increase2/1(Increase) -> Logical Operator/1
  Logical Operator1/1 -> Logical Operator2/3

== system SpeedControlTest_vDemo_TC/Validation Functions/R1 Speed Control step response/Complete step & CC active + no target & Speed Control active/Complete step detection/Step detection reset ==
  Step : Inport
  Step response : Inport  Port=2
  Active if signals constant for some specified time : Subsystem
  Logical Operator : Logic  AllPortsSameDT=off  OutDataTypeMode=Boolean
  Memory : Memory
  Step detection : Subsystem  TreatAsAtomicUnit=on  mask(Feature extraction block){StepSize=10}
      mask prompts: StepSize "Minimum step size"
      mask help: Detect a step in the signal. The minimum step size is defined by the user.
      mask CallbackString:
      | if str2double(get_param(gcb,'StepSize')) <= 0
      |     error(['Minimum step size (' get_param(gcb,'StepSize') ') out of range. Please give a value greater than zero.']);
      | else
      |     set_param([gcb '/Min step size'],'Value',get_param(gcb,'StepSize'));
      | end
  R : Outport
  wires:
  Step/1 -> Step detection/1(Signal), Active if signals constant for some specified time/2(Signal 2)
  Active if signals constant for some specified time/1(Constant signals) -> Memory/1
  Memory/1 -> Logical Operator/1
  Step response/1 -> Active if signals constant for some specified time/1(Signal1)
  Step detection/1(Step) -> Logical Operator/2
  Logical Operator/1 -> R/1

== system SpeedControlTest_vDemo_TC/Validation Functions/R1 Speed Control step response/Complete step & CC active + no target & Speed Control active/PS/Max Delay A ==
  In1 : Inport
  Delay : Constant  Value=0
  Integer Delay : S-Function  FunctionName=sfix_udelay  Parameters=samptime,vinit,NumDelays,1,1,0  mask(Integer Delay){vinit=0.0, samptime=-1, NumDelays=15}
      mask prompts: vinit "Initial condition:"; samptime "Sample time:"; NumDelays "Number of delays:"
      mask help: Delay a signal N sample periods.
      mask init:
      | if isempty(NumDelays)
      |    NumDelays = 1;
      | end
      mask Display: fprintf(' %d\nZ   ',-1*(NumDelays))
  Switch : Switch  Criteria=u2 ~= 0
  Out1 : Outport
  wires:
  Switch/1 -> Out1/1
  In1/1 -> Switch/3, Integer Delay/1
  Delay/1 -> Switch/2
  Integer Delay/1 -> Switch/1

== system SpeedControlTest_vDemo_TC/Validation Functions/R1 Speed Control step response/Complete step & CC active + no target & Speed Control active/PS/Max Delay R ==
  In1 : Inport
  Delay : Constant  Value=0
  Integer Delay : S-Function  FunctionName=sfix_udelay  Parameters=samptime,vinit,NumDelays,1,1,0  mask(Integer Delay){vinit=0.0, samptime=-1, NumDelays=15}
      mask prompts: vinit "Initial condition:"; samptime "Sample time:"; NumDelays "Number of delays:"
      mask help: Delay a signal N sample periods.
      mask init:
      | if isempty(NumDelays)
      |    NumDelays = 1;
      | end
      mask Display: fprintf(' %d\nZ   ',-1*(NumDelays))
  Switch : Switch  Criteria=u2 ~= 0
  Out1 : Outport
  wires:
  Switch/1 -> Out1/1
  In1/1 -> Switch/3, Integer Delay/1
  Delay/1 -> Switch/2
  Integer Delay/1 -> Switch/1

== system SpeedControlTest_vDemo_TC/Validation Functions/R1 Speed Control step response/Complete step & CC active + no target & Speed Control active/PS/Max Delay T ==
  In1 : Inport
  Delay : Constant  Value=0
  Integer Delay : S-Function  FunctionName=sfix_udelay  Parameters=samptime,vinit,NumDelays,1,1,0  mask(Integer Delay){vinit=0.0, samptime=-1, NumDelays=15}
      mask prompts: vinit "Initial condition:"; samptime "Sample time:"; NumDelays "Number of delays:"
      mask help: Delay a signal N sample periods.
      mask init:
      | if isempty(NumDelays)
      |    NumDelays = 1;
      | end
      mask Display: fprintf(' %d\nZ   ',-1*(NumDelays))
  Switch : Switch  Criteria=u2 ~= 0
  Out1 : Outport
  wires:
  Switch/1 -> Out1/1
  In1/1 -> Switch/3, Integer Delay/1
  Delay/1 -> Switch/2
  Integer Delay/1 -> Switch/1

== system SpeedControlTest_vDemo_TC/Validation Functions/R1 Speed Control step response/Complete step & CC active + no target & Speed Control active/PS/OR - AND ==
  R1 : Inport
  ANDop : Logic  AllPortsSameDT=off  OutDataTypeMode=Boolean
  ORop : Logic  Operator=OR  AllPortsSameDT=off  OutDataTypeMode=Boolean
  OR : Outport
  AND : Outport  Port=2
  wires:
  R1/1 -> ORop/1, ANDop/1, ORop/2, ANDop/2
  ORop/1 -> OR/1
  ANDop/1 -> AND/1

== system SpeedControlTest_vDemo_TC/Validation Functions/R1 Speed Control step response/Complete step & CC active + no target & Speed Control active/PS/TDD ==
  AND : Logic  AllPortsSameDT=off  OutDataTypeMode=Boolean
  One : Constant
  A : Outport
  T : Outport  Port=2
  wires:
  AND/1 -> T/1, A/1
  One/1 -> AND/1, AND/2

== system SpeedControlTest_vDemo_TC/Validation Functions/R1 Speed Control step response/Complete step & CC active + no target & Speed Control active/PS/TI ==
  A1 : Inport
  A2 : Inport  Port=2
  AND : Logic  AllPortsSameDT=off  OutDataTypeMode=Boolean
  Delays1 : Subsystem  TreatAsAtomicUnit=on  mask{Delay=0}
      mask prompts: Delay "Delay (in simulation steps) for the input signal:"
      mask init:
      | %set_param([gcb '/Discrete Transfer Fcn'],'Denominator',['[' num2str([1 zeros(1,str2double(get_param(gcb,'Delay')))]) ']']);
      mask CallbackString:
      | Delay = str2double(get_param(gcb,'Delay'));
      | if Delay < 0
      |     set_param(gcb,'Delay','0');
      |     error('Only non-negative delays are possible (causality).');
      |     set_param([gcb '/Delay'],'Value','0');
      | elseif Delay == 0
      |     set_param([gcb '/Delay'],'Value','0');
      | else
      |     set_param([gcb '/Integer Delay'],'NumDelays',num2str(Delay));
      |     set_param([gcb '/Delay'],'Value',num2str(Delay));
      | end
      mask Display: text(0.5,0.5,['z^{ ' num2str((-1)*str2double(get_param(gcb,'Delay'))) '}'],'texmode','on');
  Delays2 : Subsystem  TreatAsAtomicUnit=on  mask{Delay=0}
      mask prompts: Delay "Delay (in simulation steps) for the input signal:"
      mask init:
      | %set_param([gcb '/Discrete Transfer Fcn'],'Denominator',['[' num2str([1 zeros(1,str2double(get_param(gcb,'Delay')))]) ']']);
      mask CallbackString:
      | Delay = str2double(get_param(gcb,'Delay'));
      | if Delay < 0
      |     set_param(gcb,'Delay','0');
      |     error('Only non-negative delays are possible (causality).');
      |     set_param([gcb '/Delay'],'Value','0');
      | elseif Delay == 0
      |     set_param([gcb '/Delay'],'Value','0');
      | else
      |     set_param([gcb '/Integer Delay'],'NumDelays',num2str(Delay));
      |     set_param([gcb '/Delay'],'Value',num2str(Delay));
      | end
      mask Display: text(0.5,0.5,['z^{ ' num2str((-1)*str2double(get_param(gcb,'Delay'))) '}'],'texmode','on');
  A : Outport
  wires:
  AND/1 -> A/1
  A1/1 -> Delays1/1(In1)
  Delays1/1(Out1) -> AND/1
  A2/1 -> Delays2/1(In1)
  Delays2/1(Out1) -> AND/2

== system SpeedControlTest_vDemo_TC/Validation Functions/R1 Speed Control step response/Complete step & CC active + no target & Speed Control active/PS/TID ==
  T1 : Inport
  A1 : Inport  Port=2
  R OR : Inport  Port=3
  R AND : Inport  Port=4
  AND : Logic  AllPortsSameDT=off  OutDataTypeMode=Boolean
  AND1 : Logic  AllPortsSameDT=off  OutDataTypeMode=Boolean
  Hold R AND1 : Subsystem  TreatAsAtomicUnit=on
      mask Display: patch(-0.31+[0.4 0.46 0.46 0.54 0.54 0.6 0.6 0.55 0.55 0.45 0.45 0.4],-0.19+[0.85 0.85 0.95 0.95 0.85 0.85 0.87 0.87 0.96 0.96 0.87 0.87],[0 0 0]);
  Hold1 : Subsystem  TreatAsAtomicUnit=on
      mask Display: patch(-0.31+[0.4 0.46 0.46 0.54 0.54 0.6 0.6 0.55 0.55 0.45 0.45 0.4],-0.19+[0.85 0.85 0.95 0.95 0.85 0.85 0.87 0.87 0.96 0.96 0.87 0.87],[0 0 0]);
  Mem1 : Memory  Orientation=up
  Memory : Memory  Orientation=left
  OR 1 : Logic  Operator=OR  Inputs=4  AllPortsSameDT=off  OutDataTypeMode=Boolean
  OR1 : Logic  Operator=OR  Inputs=3  AllPortsSameDT=off  OutDataTypeMode=Boolean
  TA AND1 : Logic  AllPortsSameDT=off  OutDataTypeMode=Boolean
  A : Outport
  T : Outport  Port=2
  wires:
  AND1/1 -> OR1/1
  Hold R AND1/1("  ") -> AND1/1
  TA AND1/1 -> Hold1/2("    ")
  OR1/1 -> Hold1/1(" ")
  Hold1/1("  ") -> AND/1, AND/2
  A1/1 -> TA AND1/2
  OR 1/1 -> Hold R AND1/1(" ")
  T1/1 -> TA AND1/1, AND1/2, Mem1/1
  Mem1/1 -> OR 1/4
  R OR/1 -> OR1/2, OR 1/3
  R AND/1 -> Hold R AND1/2("    "), OR 1/2
  Memory/1 -> OR1/3, OR 1/1
  AND/1 -> Memory/1, T/1, A/1
